simulink model "Signaling_Model"  (R2020b)
settings: configuration reference "VLS_Standard_RH850_Signalling" (kept outside this file)
undefined symbols (not defined in the file): C_B_SlidingTiStepOfTheLeds, C_CieCurveGammaToPwmY, C_CieCurvePwmToGammaY, C_DefaultTiLEDsPwm, C_DrlRampTime, C_F_FadingDisableSlidingTI, C_F_RampTimeSlidingTI, C_IsDrlAutorizedInPower2, C_IsPlAutorizedInPower2, C_IsTiAutorizedInPower2, C_PlNominalPwm, C_PlOverDRL, C_TeAdbSlave, C_TickTIBlk, C_TiLEDsOff, C_TiSampleTime, N_MaxPwm, N_NumberOfTiLeds
libraries: Ramp_Library_R2017b x3, STD_Signaling_Lib x1
settings Model: DataDictionary=Signaling_Sldd_test.sldd  Creator=mtarek-a  LastModifiedBy=amohsen2
settings ConfigSetRef: SourceName=VLS_Standard_RH850_Signalling

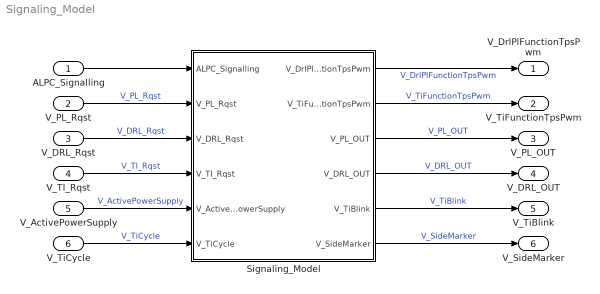
== system Signaling_Model ==
  ALPC_Signalling : Inport  OutputFunctionCall=on
  V_PL_Rqst : Inport  Port=2
  V_DRL_Rqst : Inport  Port=3
  V_TI_Rqst : Inport  Port=4
  V_ActivePowerSupply : Inport  Port=5
  V_TiCycle : Inport  Port=6
  " Signaling_Model" : Subsystem
  V_DrlPlFunctionTpsPwm : Outport
  V_TiFunctionTpsPwm : Outport  Port=2
  V_PL_OUT : Outport  Port=3
  V_DRL_OUT : Outport  Port=4
  V_TiBlink : Outport  Port=5
  V_SideMarker : Outport  Port=6
  wires:
  ALPC_Signalling/1 -> " Signaling_Model"/1(ALPC_Signalling)
  V_PL_Rqst/1 -> " Signaling_Model"/2(V_PL_Rqst)  "V_PL_Rqst"
  V_DRL_Rqst/1 -> " Signaling_Model"/3(V_DRL_Rqst)  "V_DRL_Rqst"
  V_TI_Rqst/1 -> " Signaling_Model"/4(V_TI_Rqst)  "V_TI_Rqst"
  " Signaling_Model"/1(V_DrlPlFunctionTpsPwm) -> V_DrlPlFunctionTpsPwm/1  "V_DrlPlFunctionTpsPwm"
  " Signaling_Model"/2(V_TiFunctionTpsPwm) -> V_TiFunctionTpsPwm/1  "V_TiFunctionTpsPwm"
  " Signaling_Model"/3(V_PL_OUT) -> V_PL_OUT/1  "V_PL_OUT"
  " Signaling_Model"/4(V_DRL_OUT) -> V_DRL_OUT/1  "V_DRL_OUT"
  " Signaling_Model"/5(V_TiBlink) -> V_TiBlink/1  "V_TiBlink"
  V_ActivePowerSupply/1 -> " Signaling_Model"/5(V_ActivePowerSupply)  "V_ActivePowerSupply"
  V_TiCycle/1 -> " Signaling_Model"/6(V_TiCycle)  "V_TiCycle"
  " Signaling_Model"/6(V_SideMarker) -> V_SideMarker/1  "V_SideMarker"

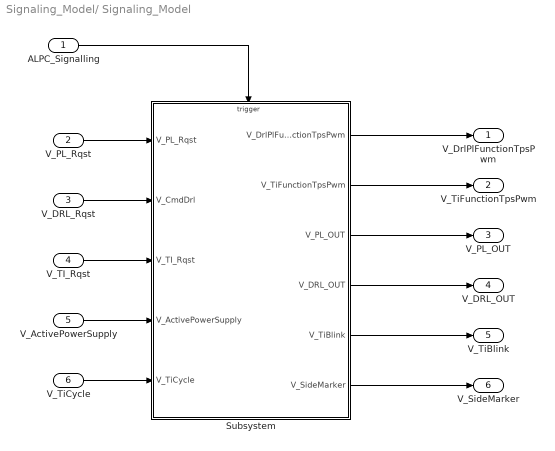
== system Signaling_Model/ Signaling_Model ==
  ALPC_Signalling : Inport  OutputFunctionCall=on
  V_PL_Rqst : Inport  Port=2
  V_DRL_Rqst : Inport  Port=3
  V_TI_Rqst : Inport  Port=4
  V_ActivePowerSupply : Inport  Port=5
  V_TiCycle : Inport  Port=6
  Subsystem : Subsystem
  V_DrlPlFunctionTpsPwm : Outport
  V_TiFunctionTpsPwm : Outport  Port=2
  V_PL_OUT : Outport  Port=3
  V_DRL_OUT : Outport  Port=4
  V_TiBlink : Outport  Port=5
  V_SideMarker : Outport  Port=6
  wires:
  V_DRL_Rqst/1 -> Subsystem/2(V_CmdDrl)
  V_TI_Rqst/1 -> Subsystem/3(V_TI_Rqst)
  Subsystem/4(V_DRL_OUT) -> V_DRL_OUT/1
  Subsystem/3(V_PL_OUT) -> V_PL_OUT/1
  Subsystem/5(V_TiBlink) -> V_TiBlink/1
  ALPC_Signalling/1 -> Subsystem/Trigger
  V_PL_Rqst/1 -> Subsystem/1(V_PL_Rqst)
  V_ActivePowerSupply/1 -> Subsystem/4(V_ActivePowerSupply)
  V_TiCycle/1 -> Subsystem/5(V_TiCycle)
  Subsystem/1(V_DrlPlFunctionTpsPwm) -> V_DrlPlFunctionTpsPwm/1
  Subsystem/2(V_TiFunctionTpsPwm) -> V_TiFunctionTpsPwm/1
  Subsystem/6(V_SideMarker) -> V_SideMarker/1

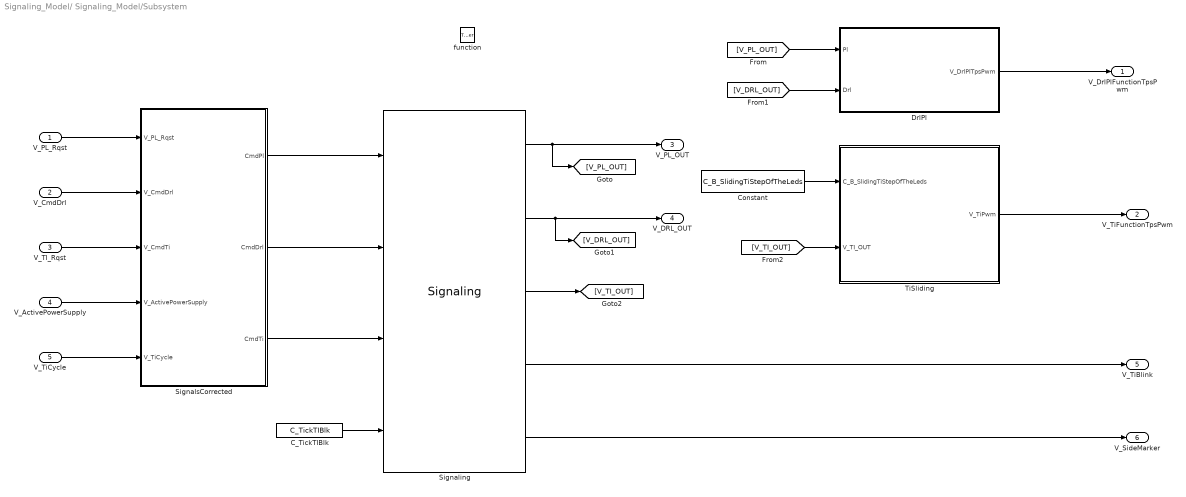
== system Signaling_Model/ Signaling_Model/Subsystem ==
  V_PL_Rqst : Inport
  V_CmdDrl : Inport  Port=2
  V_TI_Rqst : Inport  Port=3
  V_ActivePowerSupply : Inport  Port=4
  V_TiCycle : Inport  Port=5
  function : TriggerPort  TriggerType=function-call  VariantControl=Variant
  C_TickTIBlk : Constant  Value=C_TickTIBlk
  Constant : Constant  Description=|  Value=C_B_SlidingTiStepOfTheLeds
      | requirements:
      | {S___EF_286 V00}
  DrlPl : Subsystem  Description=|
      | requirements:
      | {PAMZ685_2392 V03, PAMZ685_2390 V03}
  Signaling : STD_Signaling_Lib/Signaling  SystemSampleTime=-1  VariantActivationTime=update diagram  Latency=0  AutoFrameSizeCalculation=off
      link override Subsystem1/Variant Subsystem/CONFIG_1: TreatAsAtomicUnit=on  VariantControl=CONFIG_1
      link override Subsystem1/Variant Subsystem/CONFIG_2: TreatAsAtomicUnit=on  VariantControl=CONFIG_2
      link override Subsystem1/Variant Subsystem/CONFIG_3: TreatAsAtomicUnit=on  VariantControl=CONFIG_3
      link override Subsystem1/Variant Subsystem/CONFIG_4: TreatAsAtomicUnit=on  VariantControl=CONFIG_4
      link override Subsystem1/Variant Subsystem/CONFIG_DEFAULT: TreatAsAtomicUnit=on  VariantControl=CONFIG_DEFAULT
  SignalsCorrected : Subsystem  Description=|
      | requirements:
      | {PAMZ685_2331 V03, PAMZ685_2332 V03, PAMZ685_2333 V03}
  TiSliding : Subsystem
  V_DrlPlFunctionTpsPwm : Outport
  V_TiFunctionTpsPwm : Outport  Port=2
  V_PL_OUT : Outport  Port=3  OutDataTypeStr=boolean
  V_DRL_OUT : Outport  Port=4  OutDataTypeStr=boolean
  V_TiBlink : Outport  Port=5
  V_SideMarker : Outport  Port=6
  wires:
  SignalsCorrected/1(CmdPl) -> Signaling/1
  SignalsCorrected/2(CmdDrl) -> Signaling/2
  SignalsCorrected/3(CmdTi) -> Signaling/3
  C_TickTIBlk/1 -> Signaling/4
  Signaling/1 -> V_PL_OUT/1, [V_PL_OUT]
  DrlPl/1(V_DrlPlTpsPwm) -> V_DrlPlFunctionTpsPwm/1
  TiSliding/1(V_TiPwm) -> V_TiFunctionTpsPwm/1
  [V_PL_OUT] -> DrlPl/1(Pl)
  [V_DRL_OUT] -> DrlPl/2(Drl)
  V_TiCycle/1 -> SignalsCorrected/5(V_TiCycle)
  V_TI_Rqst/1 -> SignalsCorrected/3(V_CmdTi)
  V_CmdDrl/1 -> SignalsCorrected/2("V_CmdDrl ")
  V_ActivePowerSupply/1 -> SignalsCorrected/4(V_ActivePowerSupply)
  V_PL_Rqst/1 -> SignalsCorrected/1(V_PL_Rqst)
  Constant/1 -> TiSliding/1(C_B_SlidingTiStepOfTheLeds)
  Signaling/2 -> V_DRL_OUT/1, [V_DRL_OUT]
  Signaling/4 -> V_TiBlink/1
  Signaling/3 -> [V_TI_OUT]
  [V_TI_OUT] -> TiSliding/2(V_TI_OUT)
  Signaling/5 -> V_SideMarker/1

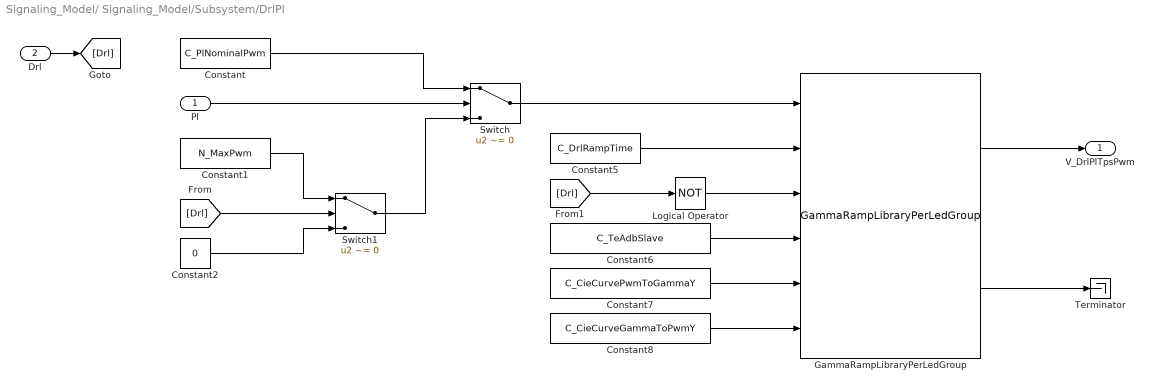
== system Signaling_Model/ Signaling_Model/Subsystem/DrlPl ==
  Pl : Inport
  Drl : Inport  Port=2
  Constant : Constant  Description=|  Value=C_PlNominalPwm
      | requirement:
      | {S___EF_274 V00 }
  Constant1 : Constant  Value=N_MaxPwm
  Constant2 : Constant  Value=0  OutDataTypeStr=Inherit: Inherit via back propagation
  Constant5 : Constant  Value=C_DrlRampTime
  Constant6 : Constant  Value=C_TeAdbSlave
  Constant7 : Constant  Value=C_CieCurvePwmToGammaY
  Constant8 : Constant  Value=C_CieCurveGammaToPwmY
  GammaRampLibraryPerLedGroup : Ramp_Library_R2017b/GammaRampLibraryPerLedGroup  Description=|  SystemSampleTime=-1  VariantActivationTime=update diagram  Latency=0  AutoFrameSizeCalculation=off
      | This library performs ramp function taking CIE curves which are evenly distributed.
      | It performs the ramp linearly on the Gamma Curve.
  Logical Operator : Logic  Operator=NOT  AllPortsSameDT=off  OutDataTypeStr=boolean
  Switch : Switch  Criteria=u2 ~= 0  OutDataTypeStr=Inherit: Inherit via back propagation
  Switch1 : Switch  Criteria=u2 ~= 0  OutDataTypeStr=Inherit: Inherit via back propagation
  Terminator : Terminator
  V_DrlPlTpsPwm : Outport
  wires:
  Switch/1 -> GammaRampLibraryPerLedGroup/1
  [Drl] -> Switch1/2
  Constant8/1 -> GammaRampLibraryPerLedGroup/6
  Constant1/1 -> Switch1/1
  Constant7/1 -> GammaRampLibraryPerLedGroup/5
  Drl/1 -> [Drl]
  Switch1/1 -> Switch/3
  Constant/1 -> Switch/1
  Constant5/1 -> GammaRampLibraryPerLedGroup/2
  [Drl] -> Logical Operator/1
  Constant6/1 -> GammaRampLibraryPerLedGroup/4
  Logical Operator/1 -> GammaRampLibraryPerLedGroup/3
  Constant2/1 -> Switch1/3
  Pl/1 -> Switch/2
  GammaRampLibraryPerLedGroup/2 -> Terminator/1
  GammaRampLibraryPerLedGroup/1 -> V_DrlPlTpsPwm/1

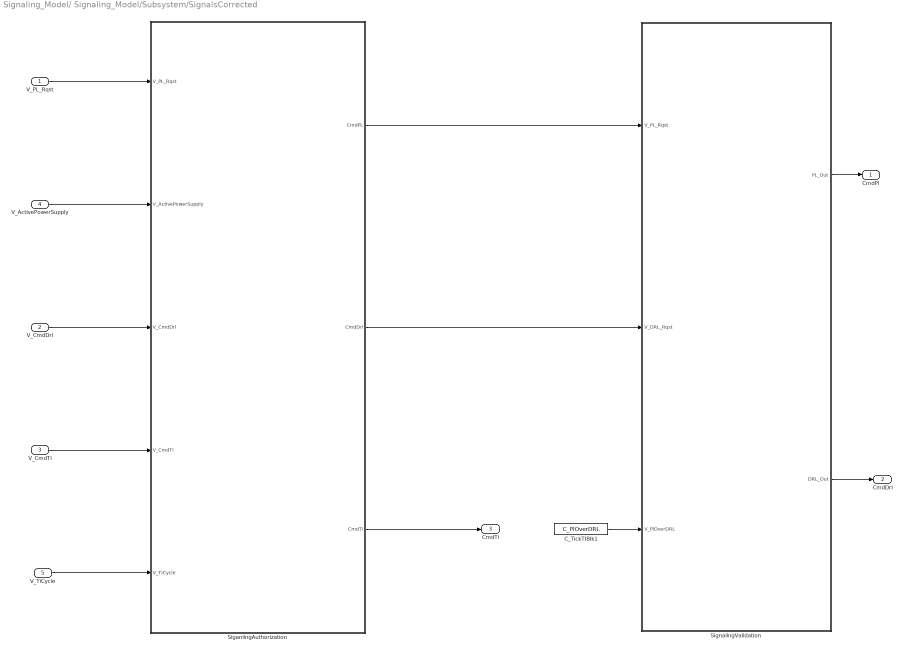
== system Signaling_Model/ Signaling_Model/Subsystem/SignalsCorrected ==
  V_PL_Rqst : Inport
  "V_CmdDrl " : Inport  Port=2
  V_CmdTi : Inport  Port=3
  V_ActivePowerSupply : Inport  Port=4
  V_TiCycle : Inport  Port=5
  C_TickTIBlk1 : Constant  Value=C_PlOverDRL
  SiganlingAuthorization : Subsystem
  SignalingValidation : Subsystem
  CmdPl : Outport
  CmdDrl : Outport  Port=2
  CmdTi : Outport  Port=3
  wires:
  SignalingValidation/2(DRL_Out) -> CmdDrl/1
  SignalingValidation/1(PL_Out) -> CmdPl/1
  C_TickTIBlk1/1 -> SignalingValidation/3(V_PlOverDRL)
  V_PL_Rqst/1 -> SiganlingAuthorization/1(V_PL_Rqst)
  V_ActivePowerSupply/1 -> SiganlingAuthorization/2(V_ActivePowerSupply)
  "V_CmdDrl "/1 -> SiganlingAuthorization/3(V_CmdDrl)
  V_CmdTi/1 -> SiganlingAuthorization/4(V_CmdTi)
  V_TiCycle/1 -> SiganlingAuthorization/5(V_TiCycle)
  SiganlingAuthorization/1(CmdPL) -> SignalingValidation/1(V_PL_Rqst)
  SiganlingAuthorization/2(CmdDrl) -> SignalingValidation/2(V_DRL_Rqst)
  SiganlingAuthorization/3(CmdTi) -> CmdTi/1

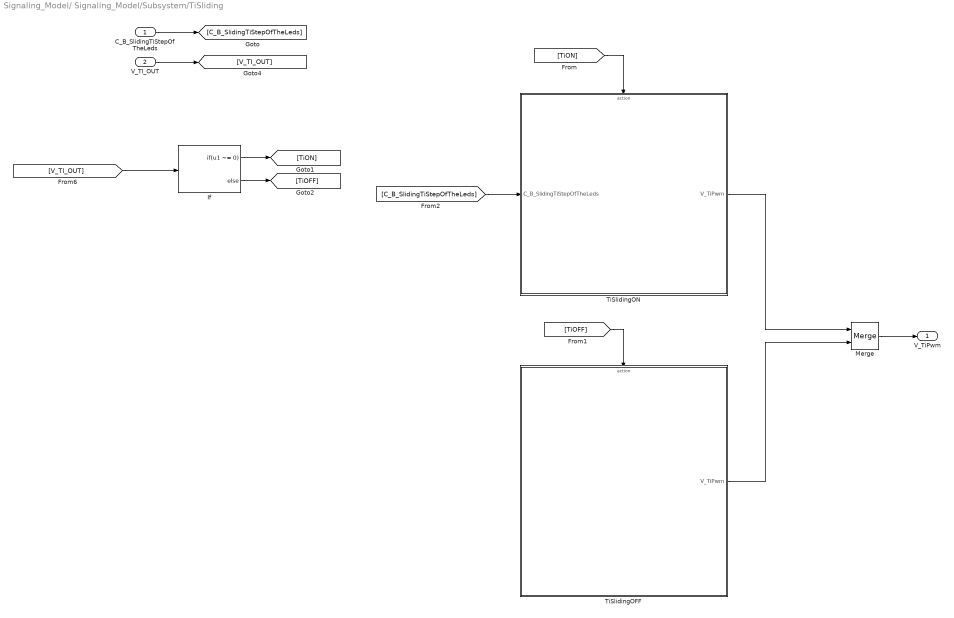
== system Signaling_Model/ Signaling_Model/Subsystem/TiSliding ==
  C_B_SlidingTiStepOfTheLeds : Inport
  V_TI_OUT : Inport  Port=2
  If : If  IfExpression=u1 ~= 0
  Merge : Merge
  TiSlidingOFF : Subsystem  TreatAsAtomicUnit=on
  TiSlidingON : Subsystem  TreatAsAtomicUnit=on
  V_TiPwm : Outport
  wires:
  C_B_SlidingTiStepOfTheLeds/1 -> [C_B_SlidingTiStepOfTheLeds]
  [TiON] -> TiSlidingON/Action
  [V_TI_OUT] -> If/1
  If/1 -> [TiON]
  If/2 -> [TiOFF]
  [TiOFF] -> TiSlidingOFF/Action
  TiSlidingOFF/1(V_TiPwm) -> Merge/2
  [C_B_SlidingTiStepOfTheLeds] -> TiSlidingON/1(C_B_SlidingTiStepOfTheLeds)
  V_TI_OUT/1 -> [V_TI_OUT]
  TiSlidingON/1(V_TiPwm) -> Merge/1
  Merge/1 -> V_TiPwm/1

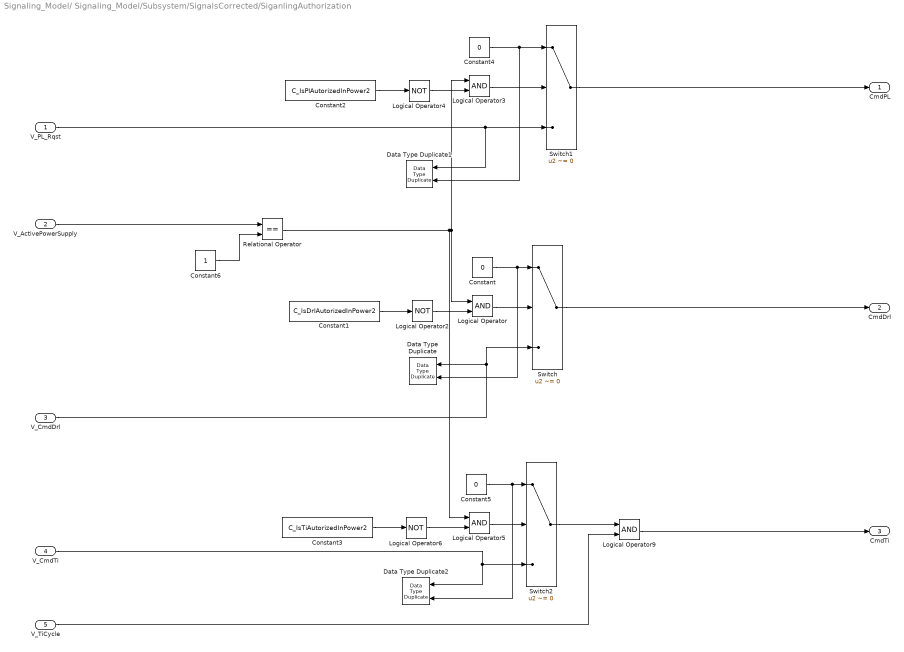
== system Signaling_Model/ Signaling_Model/Subsystem/SignalsCorrected/SiganlingAuthorization ==
  V_PL_Rqst : Inport
  V_ActivePowerSupply : Inport  Port=2
  V_CmdDrl : Inport  Port=3
  V_CmdTi : Inport  Port=4
  V_TiCycle : Inport  Port=5
  Constant : Constant  Value=0  OutDataTypeStr=Inherit: Inherit via back propagation
  Constant1 : Constant  Value=C_IsDrlAutorizedInPower2
  Constant2 : Constant  Value=C_IsPlAutorizedInPower2
  Constant3 : Constant  Value=C_IsTiAutorizedInPower2
  Constant4 : Constant  Value=0  OutDataTypeStr=Inherit: Inherit via back propagation
  Constant5 : Constant  Value=0  OutDataTypeStr=Inherit: Inherit via back propagation
  Constant6 : Constant  OutDataTypeStr=Inherit: Inherit via back propagation
  Data Type Duplicate : DataTypeDuplicate
  Data Type Duplicate1 : DataTypeDuplicate
  Data Type Duplicate2 : DataTypeDuplicate
  Logical Operator{,3,5,9} (4 alike) : Logic  AllPortsSameDT=off  OutDataTypeStr=boolean
  Logical Operator2 : Logic  Operator=NOT  AllPortsSameDT=off  OutDataTypeStr=boolean
  Logical Operator4 : Logic  Operator=NOT  AllPortsSameDT=off  OutDataTypeStr=boolean
  Logical Operator6 : Logic  Operator=NOT  AllPortsSameDT=off  OutDataTypeStr=boolean
  Relational Operator : RelationalOperator  Operator===  OutDataTypeStr=boolean  RndMeth=Simplest
  Switch : Switch  Criteria=u2 ~= 0  OutDataTypeStr=Inherit: Inherit via back propagation
  Switch1 : Switch  Criteria=u2 ~= 0  OutDataTypeStr=Inherit: Inherit via back propagation
  Switch2 : Switch  Criteria=u2 ~= 0  OutDataTypeStr=Inherit: Inherit via back propagation
  CmdPL : Outport
  CmdDrl : Outport  Port=2
  CmdTi : Outport  Port=3
  wires:
  V_CmdDrl/1 -> Switch/3, Data Type Duplicate/1
  V_PL_Rqst/1 -> Data Type Duplicate1/1, Switch1/3
  Constant6/1 -> Relational Operator/2
  Logical Operator6/1 -> Logical Operator5/2
  Constant3/1 -> Logical Operator6/1
  Logical Operator4/1 -> Logical Operator3/2
  Switch2/1 -> Logical Operator9/1
  Constant2/1 -> Logical Operator4/1
  V_CmdTi/1 -> Data Type Duplicate2/1, Switch2/3
  Relational Operator/1 -> Logical Operator3/1, Logical Operator/1, Logical Operator5/1
  Constant4/1 -> Data Type Duplicate1/2, Switch1/1
  Constant5/1 -> Data Type Duplicate2/2, Switch2/1
  Logical Operator5/1 -> Switch2/2
  Constant1/1 -> Logical Operator2/1
  Switch/1 -> CmdDrl/1
  Logical Operator3/1 -> Switch1/2
  Constant/1 -> Data Type Duplicate/2, Switch/1
  Logical Operator/1 -> Switch/2
  Logical Operator2/1 -> Logical Operator/2
  Logical Operator9/1 -> CmdTi/1
  V_TiCycle/1 -> Logical Operator9/2
  V_ActivePowerSupply/1 -> Relational Operator/1
  Switch1/1 -> CmdPL/1

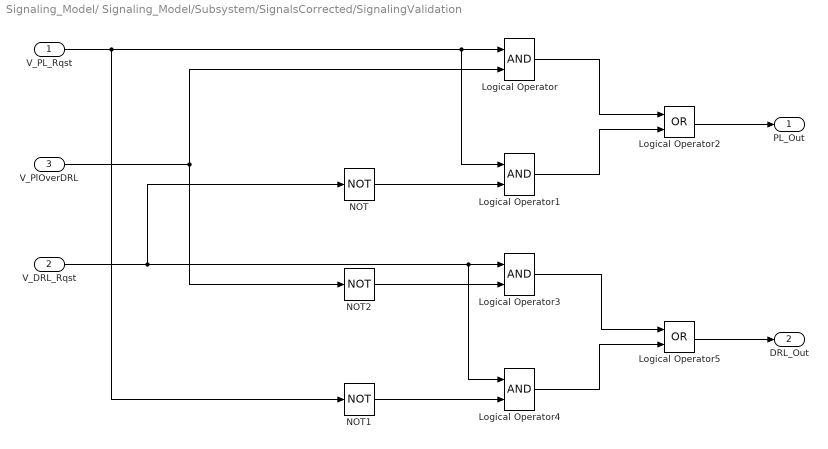
== system Signaling_Model/ Signaling_Model/Subsystem/SignalsCorrected/SignalingValidation ==
  V_PL_Rqst : Inport
  V_DRL_Rqst : Inport  Port=2
  V_PlOverDRL : Inport  Port=3
  Logical Operator{,1,3..4} (4 alike) : Logic  AllPortsSameDT=off  OutDataTypeStr=boolean
  Logical Operator2 : Logic  Operator=OR  AllPortsSameDT=off  OutDataTypeStr=boolean
  Logical Operator5 : Logic  Operator=OR  AllPortsSameDT=off  OutDataTypeStr=boolean
  NOT : Logic  Operator=NOT  IconShape=distinctive  AllPortsSameDT=off  OutDataTypeStr=boolean
  NOT1 : Logic  Operator=NOT  IconShape=distinctive  AllPortsSameDT=off  OutDataTypeStr=boolean
  NOT2 : Logic  Operator=NOT  IconShape=distinctive  AllPortsSameDT=off  OutDataTypeStr=boolean
  PL_Out : Outport
  DRL_Out : Outport  Port=2
  wires:
  Logical Operator/1 -> Logical Operator2/1
  Logical Operator2/1 -> PL_Out/1
  NOT/1 -> Logical Operator1/2
  V_DRL_Rqst/1 -> NOT/1, Logical Operator4/1, Logical Operator3/1
  V_PlOverDRL/1 -> Logical Operator/2, NOT2/1
  Logical Operator5/1 -> DRL_Out/1
  NOT1/1 -> Logical Operator4/2
  Logical Operator1/1 -> Logical Operator2/2
  NOT2/1 -> Logical Operator3/2
  Logical Operator3/1 -> Logical Operator5/1
  Logical Operator4/1 -> Logical Operator5/2
  V_PL_Rqst/1 -> Logical Operator/1, Logical Operator1/1, NOT1/1

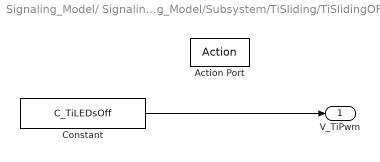
== system Signaling_Model/ Signaling_Model/Subsystem/TiSliding/TiSlidingOFF ==
  Action Port : ActionPort  ActionPortLabel=else
  Constant : Constant  Value=C_TiLEDsOff
  V_TiPwm : Outport
  wires:
  Constant/1 -> V_TiPwm/1

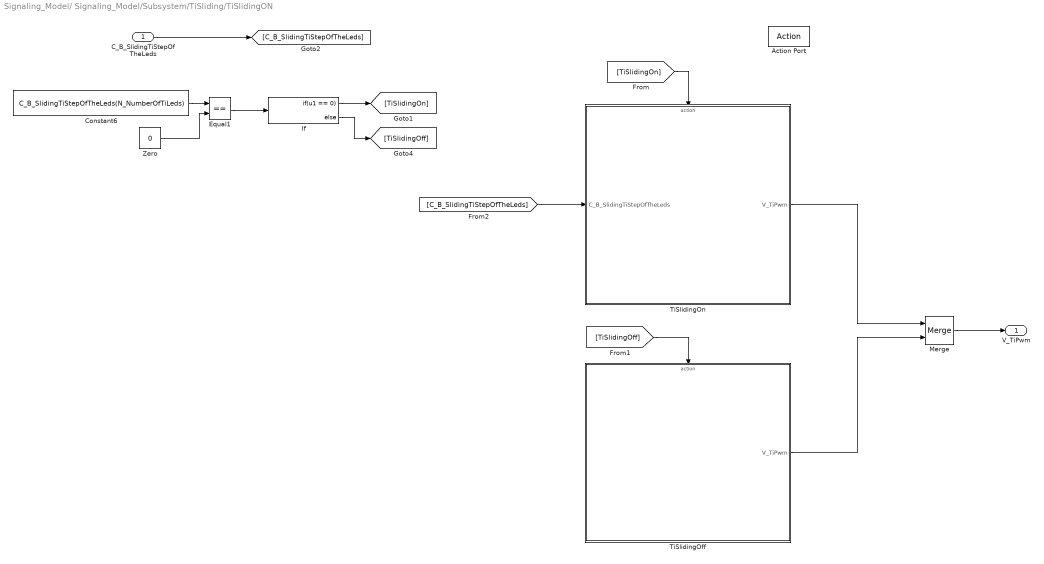
== system Signaling_Model/ Signaling_Model/Subsystem/TiSliding/TiSlidingON ==
  C_B_SlidingTiStepOfTheLeds : Inport
  Action Port : ActionPort  ActionPortLabel=if(u1 ~= 0)
  Constant6 : Constant  Value=C_B_SlidingTiStepOfTheLeds(N_NumberOfTiLeds)
  Equal1 : RelationalOperator  Operator===  OutDataTypeStr=boolean  RndMeth=Simplest
  If : If  IfExpression=u1 == 0
  Merge : Merge
  TiSlidingOff : Subsystem  Description=|  TreatAsAtomicUnit=on
      | requirements:
      | {S___EF_322 V00}
  TiSlidingOn : Subsystem  Description=|  TreatAsAtomicUnit=on
      | requirements:
      | {S___EF_284 V00, }
  Zero : Constant  Value=0  OutDataTypeStr=Inherit: Inherit via back propagation
  V_TiPwm : Outport
  wires:
  C_B_SlidingTiStepOfTheLeds/1 -> [C_B_SlidingTiStepOfTheLeds]
  Constant6/1 -> Equal1/1
  Zero/1 -> Equal1/2
  Equal1/1 -> If/1
  If/1 -> [TiSlidingOn]
  If/2 -> [TiSlidingOff]
  [TiSlidingOn] -> TiSlidingOn/Action
  [TiSlidingOff] -> TiSlidingOff/Action
  [C_B_SlidingTiStepOfTheLeds] -> TiSlidingOn/1(C_B_SlidingTiStepOfTheLeds)
  TiSlidingOn/1(V_TiPwm) -> Merge/1
  TiSlidingOff/1(V_TiPwm) -> Merge/2
  Merge/1 -> V_TiPwm/1

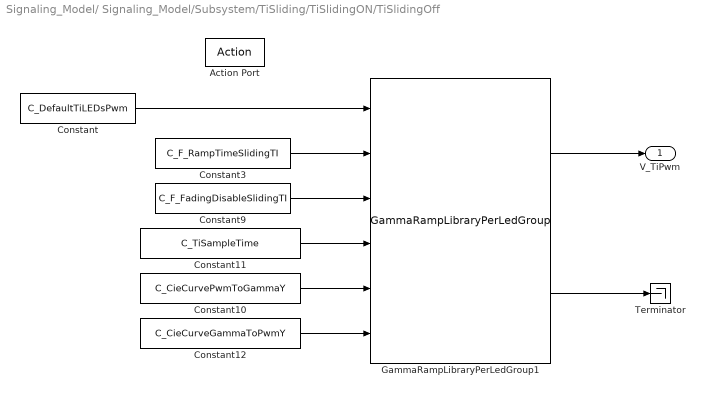
== system Signaling_Model/ Signaling_Model/Subsystem/TiSliding/TiSlidingON/TiSlidingOff ==
  Action Port : ActionPort  ActionPortLabel=else
  Constant : Constant  Value=C_DefaultTiLEDsPwm
  Constant10 : Constant  Value=C_CieCurvePwmToGammaY
  Constant11 : Constant  Value=C_TiSampleTime
  Constant12 : Constant  Value=C_CieCurveGammaToPwmY
  Constant3 : Constant  Value=C_F_RampTimeSlidingTI
  Constant9 : Constant  Value=C_F_FadingDisableSlidingTI
  GammaRampLibraryPerLedGroup1 : Ramp_Library_R2017b/GammaRampLibraryPerLedGroup  Description=|  SystemSampleTime=-1  VariantActivationTime=update diagram  Latency=0  AutoFrameSizeCalculation=off
      | This library performs ramp function taking CIE curves which are evenly distributed.
      | It performs the ramp linearly on the Gamma Curve.
  Terminator : Terminator
  V_TiPwm : Outport
  wires:
  Constant10/1 -> GammaRampLibraryPerLedGroup1/5
  GammaRampLibraryPerLedGroup1/1 -> V_TiPwm/1
  GammaRampLibraryPerLedGroup1/2 -> Terminator/1
  Constant12/1 -> GammaRampLibraryPerLedGroup1/6
  Constant11/1 -> GammaRampLibraryPerLedGroup1/4
  Constant/1 -> GammaRampLibraryPerLedGroup1/1
  Constant3/1 -> GammaRampLibraryPerLedGroup1/2
  Constant9/1 -> GammaRampLibraryPerLedGroup1/3

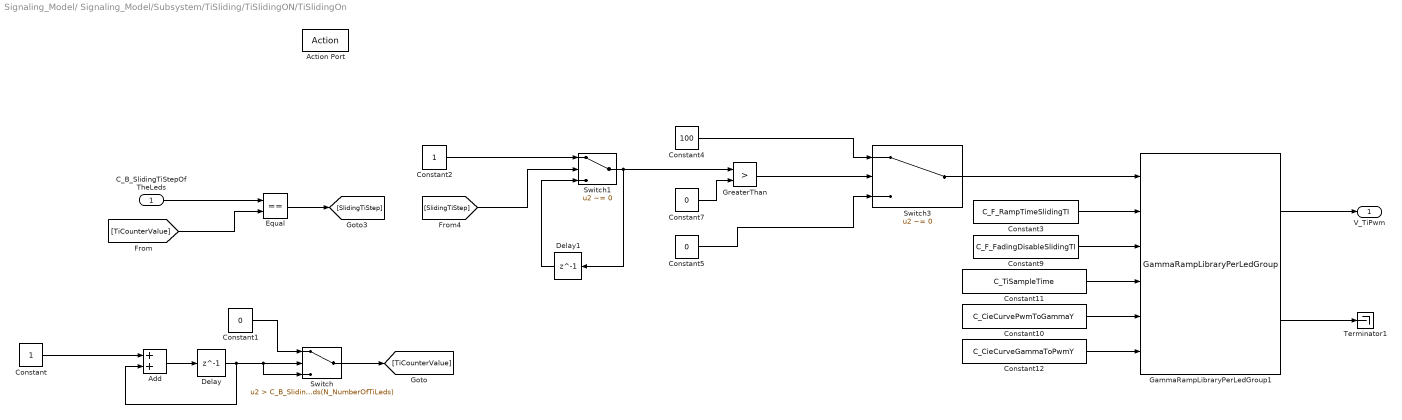
== system Signaling_Model/ Signaling_Model/Subsystem/TiSliding/TiSlidingON/TiSlidingOn ==
  C_B_SlidingTiStepOfTheLeds : Inport
  Action Port : ActionPort  ActionPortLabel=if(u1 == 0)
  Add : Sum  AccumDataTypeStr=uint8  OutDataTypeStr=uint8
  Constant : Constant  OutDataTypeStr=Inherit: Inherit via back propagation
  Constant1 : Constant  Value=0  OutDataTypeStr=Inherit: Inherit via back propagation
  Constant10 : Constant  Value=C_CieCurvePwmToGammaY
  Constant11 : Constant  Value=C_TiSampleTime
  Constant12 : Constant  Value=C_CieCurveGammaToPwmY
  Constant2 : Constant  OutDataTypeStr=Inherit: Inherit via back propagation
  Constant3 : Constant  Description=|  Value=C_F_RampTimeSlidingTI
      | requirements:
      | {S___EF_289 V00 }
  Constant4 : Constant  Value=100  OutDataTypeStr=Inherit: Inherit via back propagation
  Constant5 : Constant  Value=0  OutDataTypeStr=Inherit: Inherit via back propagation
  Constant7 : Constant  Value=0  OutDataTypeStr=Inherit: Inherit via back propagation
  Constant9 : Constant  Description=|  Value=C_F_FadingDisableSlidingTI
      | requirements:
      | {S___EF_292 V00 }
  Delay : Delay  DelayLength=1
  Delay1 : Delay  DelayLength=1
  Equal : RelationalOperator  Operator===  OutDataTypeStr=boolean  RndMeth=Simplest
  GammaRampLibraryPerLedGroup1 : Ramp_Library_R2017b/GammaRampLibraryPerLedGroup  Description=|  SystemSampleTime=-1  VariantActivationTime=update diagram  Latency=0  AutoFrameSizeCalculation=off
      | requirements:
      | {S___EF_290 V00, S___EF_291 V00}
  GreaterThan : RelationalOperator  Operator=>  OutDataTypeStr=boolean  RndMeth=Simplest
  Switch : Switch  Description=|  Criteria=u2 > Threshold  Threshold=C_B_SlidingTiStepOfTheLeds(N_NumberOfTiLeds)
      | requirements:
      | {S___EF_288 V00 }
  Switch1 : Switch  Criteria=u2 ~= 0  OutDataTypeStr=uint8
  Switch3 : Switch  Criteria=u2 ~= 0  OutDataTypeStr=fixdt(0,16,0.01,0)
  Terminator1 : Terminator
  V_TiPwm : Outport
  wires:
  Delay/1 -> Add/2, Switch/3, Switch/2
  Constant11/1 -> GammaRampLibraryPerLedGroup1/4
  Constant3/1 -> GammaRampLibraryPerLedGroup1/2
  GammaRampLibraryPerLedGroup1/2 -> Terminator1/1
  Constant12/1 -> GammaRampLibraryPerLedGroup1/6
  Constant9/1 -> GammaRampLibraryPerLedGroup1/3
  GammaRampLibraryPerLedGroup1/1 -> V_TiPwm/1
  Constant7/1 -> GreaterThan/2
  Constant10/1 -> GammaRampLibraryPerLedGroup1/5
  Switch3/1 -> GammaRampLibraryPerLedGroup1/1
  Constant4/1 -> Switch3/1
  Switch/1 -> [TiCounterValue]
  Constant/1 -> Add/1
  Constant1/1 -> Switch/1
  Switch1/1 -> Delay1/1, GreaterThan/1
  Add/1 -> Delay/1
  [TiCounterValue] -> Equal/2
  C_B_SlidingTiStepOfTheLeds/1 -> Equal/1
  Delay1/1 -> Switch1/3
  GreaterThan/1 -> Switch3/2
  Constant2/1 -> Switch1/1
  Equal/1 -> [SlidingTiStep]
  [SlidingTiStep] -> Switch1/2
  Constant5/1 -> Switch3/3
